simulink model "simulazione_simulink_punto3"  (R2023a)
settings: Solver=VariableStepAuto  StartTime=0.0  StopTime=100  RelTol=1e-3
values from neighbouring files (symbols this model uses):
  A = [0,0,1,0 ; 0,0,0,1 ; -k/m1, k/m1, -c/m1, c/m1 ; k/m2, -k/m2, c/m2, -c/m2]    [Compito4.m]
  B = [0 ; 0 ; 1/m1 ; 0]    [Compito4.m]
  C = [1, 0, 0, 0]    [Compito4.m]
  D = 0    [Compito4.m]
  F = -place(A,B,poles)    [Compito4.m]
  g1 = 0    [Compito4.m]
  g2 = 0    [Compito4.m]
  g3 = 10    [Compito4.m]
  g4 = 0    [Compito4.m]
  L = 3    [Compito4.m]
  V = -Fd'    [Compito4.m]
  x_0 = [0 ; 0 ; 0 ; 0]    [Compito4.m]
libraries: simulink x1
settings Model: Creator=Valeria  LastModifiedBy=simon

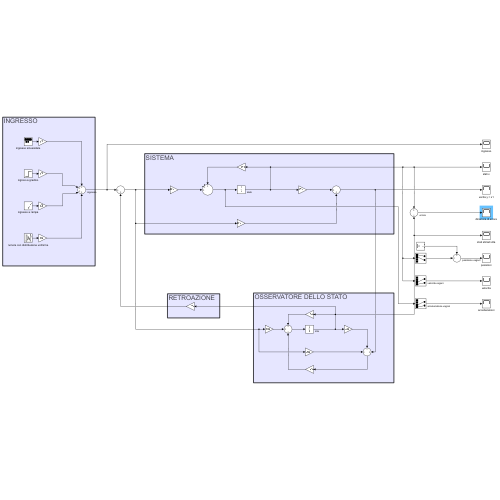
[thumbnail: Simulink's stored preview of the top-level diagram]
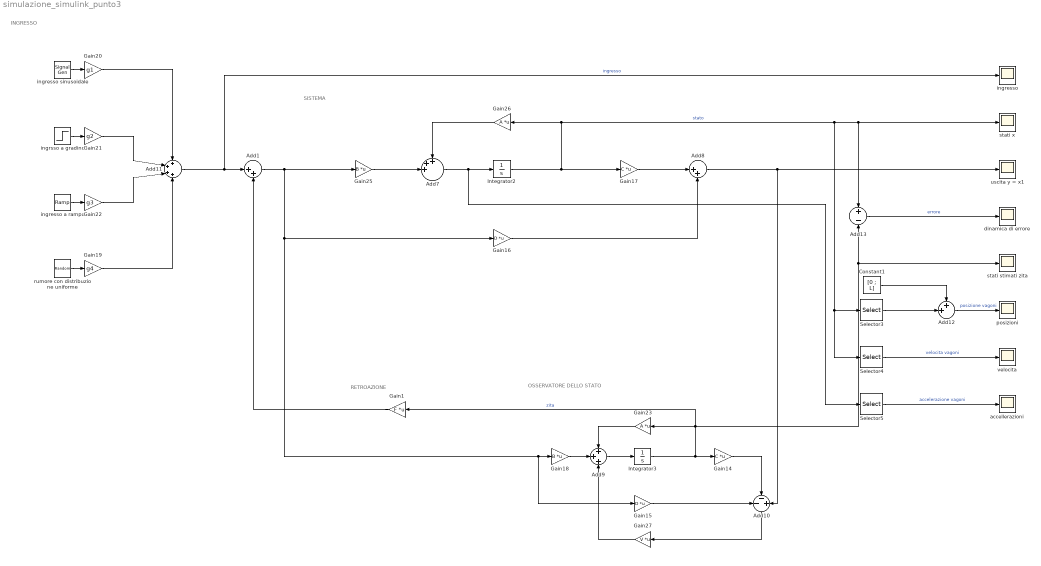
== system simulazione_simulink_punto3 ==
  note: RETROAZIONE
  note: SISTEMA
  note: OSSERVATORE DELLO STATO
  note: INGRESSO
  Add1 : Sum  Inputs=|++
  Add10 : Sum  Inputs=--+
  Add11 : Sum  Inputs=++++
  Add12 : Sum  Inputs=++|
  Add13 : Sum  Inputs=+-
  Add7 : Sum  Inputs=+++||
  Add8 : Sum  Inputs=|++
  Add9 : Sum  Inputs=+++
  Constant1 : Constant  Value=[0 ; L]
  Gain1 : Gain  Gain=F  Multiplication=Matrix(K*u)
  Gain14 : Gain  Gain=C  Multiplication=Matrix(K*u)
  Gain15 : Gain  Gain=D  Multiplication=Matrix(K*u)
  Gain16 : Gain  Gain=D  Multiplication=Matrix(K*u)
  Gain17 : Gain  Gain=C  Multiplication=Matrix(K*u)
  Gain18 : Gain  Gain=B  Multiplication=Matrix(K*u)
  Gain19 : Gain  Gain=g4
  Gain20 : Gain  Gain=g1
  Gain21 : Gain  Gain=g2
  Gain22 : Gain  Gain=g3
  Gain23 : Gain  Gain=A  Multiplication=Matrix(K*u)
  Gain25 : Gain  Gain=B  Multiplication=Matrix(K*u)
  Gain26 : Gain  Gain=A  Multiplication=Matrix(K*u)
  Gain27 : Gain  Gain=V  Multiplication=Matrix(K*u)
  Integrator2 : Integrator  InitialCondition=x_0
  Integrator3 : Integrator
  Selector3 : Selector  InputPortWidth=4  IndexOptions=Index vector (dialog)  Indices=[1 2]  OutputSizes=1  RuntimeRangeChecks=on
  Selector4 : Selector  InputPortWidth=4  IndexOptions=Index vector (dialog)  Indices=[3 4]  OutputSizes=1  RuntimeRangeChecks=on
  Selector5 : Selector  InputPortWidth=4  IndexOptions=Index vector (dialog)  Indices=[3 4]  OutputSizes=1  RuntimeRangeChecks=on
  accellerazioni : Scope
  dinamica di errore : Scope
  ingresso : Scope
  ingresso a rampa : simulink/Sources/Ramp  slope=1  start=0  InitialOutput=0
  ingresso sinusoidale : SignalGenerator
  ingrsso a gradino : Step  Time=0  SampleTime=0  ZeroCross=off
  posizioni : Scope
  rumore con distribuzione uniforme : UniformRandomNumber  SampleTime=0.1
  stati stimati zita : Scope
  stati x : Scope
  uscita y = x1 : Scope
  velocita : Scope
  wires:
  Selector3/1 -> Add12/2
  Add12/1 -> posizioni/1  "posizione vagoni"
  Gain19/1 -> Add11/4
  ingrsso a gradino/1 -> Gain21/1
  Add7/1 -> Selector5/1, Integrator2/1
  Gain23/1 -> Add9/1
  Add10/1 -> Gain27/1
  Gain27/1 -> Add9/3
  Gain25/1 -> Add7/3
  Integrator3/1 -> Gain1/1, Gain23/1, Add13/2, stati stimati zita/1, Gain14/1  "zita"
  Add9/1 -> Integrator3/1
  Gain26/1 -> Add7/1
  Gain16/1 -> Add8/2
  ingresso a rampa/1 -> Gain22/1
  Gain21/1 -> Add11/2
  ingresso sinusoidale/1 -> Gain20/1
  Gain14/1 -> Add10/2
  Add8/1 -> Add10/3, uscita y = x1/1
  Integrator2/1 -> Gain17/1, Selector3/1, Selector4/1, stati x/1, Add13/1, Gain26/1  "stato"
  Gain20/1 -> Add11/1
  Gain18/1 -> Add9/2
  rumore con distribuzione uniforme/1 -> Gain19/1
  Gain15/1 -> Add10/1
  Selector4/1 -> velocita/1  "velocita vagoni"
  Gain17/1 -> Add8/1
  Add13/1 -> dinamica di errore/1  "errore"
  Constant1/1 -> Add12/1
  Gain22/1 -> Add11/3
  Selector5/1 -> accellerazioni/1  "accelerazione vagoni"
  Add11/1 -> ingresso/1, Add1/1  "ingresso"
  Gain1/1 -> Add1/2
  Add1/1 -> Gain25/1, Gain16/1, Gain15/1, Gain18/1
